simulink model "Controller"  (R2015a)
settings: Solver=ode3  SolverMode=SingleTasking  StartTime=0.0  StopTime=100  FixedStep=T_sim  RelTol=1e-3
PreLoadFcn:
  | LoadLibraries
values from neighbouring files (symbols this model uses):
  a = 10.26    [SetupComplete.m]
  A_x = 0.015    [SetupComplete.m]
  A_y = A_x    (= 0.015)    [SetupComplete.m]
  A_z = 0.16    [SetupComplete.m]
  C_d0 = 0.001193    [SetupComplete.m]
  C_x = 1.2    [SetupComplete.m]
  C_y = C_x    (= 1.2)    [SetupComplete.m]
  C_z = 2.2    [SetupComplete.m]
  CG_0 = [0,0,0.02]'    [SetupComplete.m]
  eta_23 = deg2rad(-1.42)    [Run3Copter.m]
  g = 9.81    [SetupComplete.m]
  h = 0.08    [SetupComplete.m]
  h_M = 0.064    [SetupComplete.m]
  I_BAC_0 = [ Ix,0,Ixz;0,Iy,0;Ixz,0,Iz]    [SetupComplete.m]
  Initial_Omegas = [1;1;1]*Omega_hover    [Run3Copter.m]
  l = 0.3450    (= 0.345)    [NDI_components.m]    (also in SetupComplete.m; robust_controller.m)
  l_arm = 0.264    [SetupComplete.m]
  m = 3.51    [SetupComplete.m]
  m_0 = 2.61    [SetupComplete.m]
  m_M = 0.300    (= 0.3)    [SetupComplete.m]
  R = 0.1778    [SetupComplete.m]    (also in robust_controller.m = eye(4))
  rho = 1.15    [SetupComplete.m]
  sigma = b*c/(pi*R)    (= 0.107416159567)    [SetupComplete.m]
  theta_0 = 0.38397    [SetupComplete.m]
  theta_1 = -0.2967    [SetupComplete.m]
  v_i0 = sqrt( 1/3*m*g/(2*rho*pi*R^2)  )    [SetupComplete.m]
undefined symbols (not defined in the file or in its folder): DOWN_0, EAST_0, Motor, NORTH_0, P_0, Prop, Q_0, R_0, Throttle_Hover, U_0, V_0, v_i_adim, Vx_adim, Vz_adim, W_0
undefined symbols (not defined in the file): Initial_Torques, J_FA, J_T, Rotation_sign, Tau_motors
libraries: XXCopter x39, simulink x35, vrlib x15, simulink_extras x7, aerolib6dofsys x2, qcatlib x2, dspinverses x2
(part 4 of 10)

== system Controller/P Controller/NDI+CA Controller/ 9DOF NDI+CA Controller - No massic update/1st order reference model ==
  y_ref : Inport
  y_meas : Inport  Port=2
  Bandwidth gain : Gain  Gain=Kb
  Bandwidth gain 1 : Gain  Gain=Kb
  Command FF gain : Gain  Gain=fc
  Command_dot FF gain : Gain  Gain=Kf
  Integral gain : Gain  Gain=fi
  Integrator : Integrator
  Integrator1 : Integrator
  Kref gain : Gain  Gain=Kref
  Sum15 : Sum  Inputs=|+-
  Sum16 : Sum  Inputs=++-
  Sum17 : Sum  Inputs=++|
  Sum5 : Sum  Inputs=|+-
  y_des_dot : Outport
  wires:
  Integral gain/1 -> Integrator1/1
  Bandwidth gain 1/1 -> Integral gain/1
  y_ref/1 -> Sum5/1
  Command_dot FF gain/1 -> Sum17/1
  Command FF gain/1 -> Sum16/1
  Integrator/1 -> Command FF gain/1, Sum15/1, Sum5/2  "y_c"
  y_meas/1 -> Sum16/3, Sum15/2
  Sum16/1 -> Bandwidth gain/1
  Kref gain/1 -> Integrator/1, Command_dot FF gain/1  "y_dot_c"
  Integrator1/1 -> Sum16/2
  Sum17/1 -> y_des_dot/1
  Bandwidth gain/1 -> Sum17/2
  Sum15/1 -> Bandwidth gain 1/1
  Sum5/1 -> Kref gain/1

== system Controller/P Controller/NDI+CA Controller/ 9DOF NDI+CA Controller - No massic update/Control Allocation 9DOF ==
  Pseudocontrol input : Inport
  Effectiveness control matrix : Inport  Port=2
  Control Allocation 9DOF : Subsystem  VariantControl=(default)
  Pseudoinverse 9DOF : Subsystem  VariantControl=Variant1
  Control output : Outport

== system Controller/P Controller/NDI+CA Controller/4DOF NDI+CA Controller - No massic update/1st order reference model ==
  y_ref : Inport
  y_meas : Inport  Port=2
  Bandwidth gain : Gain  Gain=Kb
  Bandwidth gain 1 : Gain  Gain=Kb
  Command FF gain : Gain  Gain=fc
  Command_dot FF gain : Gain  Gain=Kf
  Integral gain : Gain  Gain=fi
  Integrator : Integrator
  Integrator1 : Integrator
  Kref gain : Gain  Gain=Kref
  Sum15 : Sum  Inputs=|+-
  Sum16 : Sum  Inputs=++-
  Sum17 : Sum  Inputs=++|
  Sum5 : Sum  Inputs=|+-
  y_des_dot : Outport
  wires:
  Sum5/1 -> Kref gain/1
  Sum15/1 -> Bandwidth gain 1/1
  Bandwidth gain/1 -> Sum17/2
  Sum17/1 -> y_des_dot/1
  Integrator1/1 -> Sum16/2
  Kref gain/1 -> Command_dot FF gain/1, Integrator/1  "y_dot_c"
  Sum16/1 -> Bandwidth gain/1
  y_meas/1 -> Sum15/2, Sum16/3
  Integrator/1 -> Sum5/2, Sum15/1, Command FF gain/1  "y_c"
  Command FF gain/1 -> Sum16/1
  Command_dot FF gain/1 -> Sum17/1
  y_ref/1 -> Sum5/1
  Bandwidth gain 1/1 -> Integral gain/1
  Integral gain/1 -> Integrator1/1

== system Controller/P Controller/NDI+CA Controller/4DOF NDI+CA Controller - No massic update/1st order reference model1 ==
  y_ref : Inport
  y_meas : Inport  Port=2
  Bandwidth gain : Gain  Gain=Kb
  Bandwidth gain 1 : Gain  Gain=Kb
  Command FF gain : Gain  Gain=fc
  Command_dot FF gain : Gain  Gain=Kf
  Integral gain : Gain  Gain=fi
  Integrator : Integrator
  Integrator1 : Integrator
  Kref gain : Gain  Gain=Kref
  Sum15 : Sum  Inputs=|+-
  Sum16 : Sum  Inputs=++-
  Sum17 : Sum  Inputs=++|
  Sum5 : Sum  Inputs=|+-
  y_des_dot : Outport
  wires:
  Sum5/1 -> Kref gain/1
  Sum15/1 -> Bandwidth gain 1/1
  Bandwidth gain/1 -> Sum17/2
  Sum17/1 -> y_des_dot/1
  Integrator1/1 -> Sum16/2
  Kref gain/1 -> Command_dot FF gain/1, Integrator/1  "y_dot_c"
  Sum16/1 -> Bandwidth gain/1
  y_meas/1 -> Sum15/2, Sum16/3
  Integrator/1 -> Sum5/2, Sum15/1, Command FF gain/1  "y_c"
  Command FF gain/1 -> Sum16/1
  Command_dot FF gain/1 -> Sum17/1
  y_ref/1 -> Sum5/1
  Bandwidth gain 1/1 -> Integral gain/1
  Integral gain/1 -> Integrator1/1

== system Controller/P Controller/NDI+CA Controller/4DOF NDI+CA Controller - No massic update/1st order reference model2 ==
  y_ref : Inport
  y_meas : Inport  Port=2
  Bandwidth gain : Gain  Gain=Kb
  Bandwidth gain 1 : Gain  Gain=Kb
  Command FF gain : Gain  Gain=fc
  Command_dot FF gain : Gain  Gain=Kf
  Integral gain : Gain  Gain=fi
  Integrator : Integrator
  Integrator1 : Integrator
  Kref gain : Gain  Gain=Kref
  Sum15 : Sum  Inputs=|+-
  Sum16 : Sum  Inputs=++-
  Sum17 : Sum  Inputs=++|
  Sum5 : Sum  Inputs=|+-
  y_des_dot : Outport
  wires:
  Sum5/1 -> Kref gain/1
  Sum15/1 -> Bandwidth gain 1/1
  Bandwidth gain/1 -> Sum17/2
  Sum17/1 -> y_des_dot/1
  Integrator1/1 -> Sum16/2
  Kref gain/1 -> Command_dot FF gain/1, Integrator/1  "y_dot_c"
  Sum16/1 -> Bandwidth gain/1
  y_meas/1 -> Sum15/2, Sum16/3
  Integrator/1 -> Sum5/2, Sum15/1, Command FF gain/1  "y_c"
  Command FF gain/1 -> Sum16/1
  Command_dot FF gain/1 -> Sum17/1
  y_ref/1 -> Sum5/1
  Bandwidth gain 1/1 -> Integral gain/1
  Integral gain/1 -> Integrator1/1

== system Controller/P Controller/NDI+CA Controller/4DOF NDI+CA Controller - No massic update/1st order reference model3 ==
  y_ref : Inport
  y_meas : Inport  Port=2
  Bandwidth gain : Gain  Gain=Kb
  Bandwidth gain 1 : Gain  Gain=Kb
  Command FF gain : Gain  Gain=fc
  Command_dot FF gain : Gain  Gain=Kf
  Integral gain : Gain  Gain=fi
  Integrator : Integrator
  Integrator1 : Integrator
  Kref gain : Gain  Gain=Kref
  Sum15 : Sum  Inputs=|+-
  Sum16 : Sum  Inputs=++-
  Sum17 : Sum  Inputs=++|
  Sum5 : Sum  Inputs=|+-
  y_des_dot : Outport
  wires:
  Integral gain/1 -> Integrator1/1
  Bandwidth gain 1/1 -> Integral gain/1
  y_ref/1 -> Sum5/1
  Command_dot FF gain/1 -> Sum17/1
  Command FF gain/1 -> Sum16/1
  Integrator/1 -> Command FF gain/1, Sum15/1, Sum5/2  "y_c"
  y_meas/1 -> Sum16/3, Sum15/2
  Sum16/1 -> Bandwidth gain/1
  Kref gain/1 -> Integrator/1, Command_dot FF gain/1  "y_dot_c"
  Integrator1/1 -> Sum16/2
  Sum17/1 -> y_des_dot/1
  Bandwidth gain/1 -> Sum17/2
  Sum15/1 -> Bandwidth gain 1/1
  Sum5/1 -> Kref gain/1

== system Controller/P Controller/NDI+CA Controller/4DOF NDI+CA Controller - No massic update/Control Allocation 4DOF ==
  Pseudocontrol input : Inport
  Effectiveness control matrix : Inport  Port=2
  Control Allocation 4DOF : Subsystem  VariantControl=(default)
  Pseudoinverse : Subsystem  VariantControl=Variant1
  Control output : Outport

== system Controller/P Controller/NDI+CA Controller/9DOF NDI+CA Controller/Mass Properties ==
  Arms DCMs : Inport
  CG_0 : Inport  Port=2
  m_0 : Inport  Port=3
  m : Inport  Port=4
  m_M : Inport  Port=5
  I_BAC_0 : Inport  Port=6
  Arm Inertia : MATLAB Function  TreatAsAtomicUnit=on
  Bus Selector : BusSelector  OutputSignals=T_FaFb1,T_FaFb2,T_FaFb3
  CG position : Sum
  Divide : Product  Inputs=*/
  Divide1 : Product  Inputs=**
  Divide2 : Product  Inputs=/*
  Divide3 : Product  Inputs=**
  Motors Pos sum : Sum  Inputs=+++
  Total I_BAC : Sum
  I_BAC : Outport
  CG : Outport  Port=2
  wires:
  Arms DCMs/1 -> Bus Selector/1
  Bus Selector/3 -> Arm Inertia/3(T3_FAFb)  "<T_FaFb3>"
  Bus Selector/2 -> Arm Inertia/2(T2_FAFb)  "<T_FaFb2>"
  Bus Selector/1 -> Arm Inertia/1(T1_FAFb)  "<T_FaFb1>"
  Total I_BAC/1 -> I_BAC/1
  m_0/1 -> Divide/1
  m/1 -> Divide/2, Divide2/1
  CG_0/1 -> Divide1/1
  Divide/1 -> Divide1/2
  m_M/1 -> Divide2/2
  CG position/1 -> CG/1
  Divide1/1 -> CG position/1
  Motors Pos sum/1 -> Divide3/1
  Divide2/1 -> Divide3/2
  Divide3/1 -> CG position/2
  Arm Inertia/3(r2_M) -> Motors Pos sum/2
  Arm Inertia/4(r3_M) -> Motors Pos sum/1
  Arm Inertia/1(I_M) -> Total I_BAC/2
  I_BAC_0/1 -> Total I_BAC/1
  Arm Inertia/2(r1_M) -> Motors Pos sum/3

== system Controller/3 Copter Complete/Arms Dynamics: Forces and Moments/4 DOF Arms Dynamics: Forces and Moments1/4 DOF Arms Dynamics: Forces and Moments1/Arm Dynamics ==
  note: Motor-Propeller Coupling: Propeller Torque
  Throttle [0-1] : Inport
  Comm Angles (rad) : Inport  Port=2
  Omega_Initial : Inport  Port=3
  h_ground : Inport  Port=4
  omega_b : Inport  Port=5
  V_b : Inport  Port=6
  Aerodynamics Propeller : Subsystem  TreatAsAtomicUnit=on  mask{Rot_sign=Rot_sign}
      mask prompts: Rot_sign "Rotation Sign"
      settings: MinAlgLoopOccurrences=on
      mask TypeOptions Rot_sign: Rotation_sign/Value
  Arms Kinematics : Subsystem  AncestorBlock=XXCopter/Arms Kinematics  TreatAsAtomicUnit=on  mask{Arm_number=arm_num, Arm_hub_position=arm_hub_pos, eta_dir=eta_dir, gamma_dir=gamma_dir, h_prop=h}
      mask prompts: Arm_number "Arm number (1,2 or 3)"; Arm_hub_position "Arm Hub position"; eta_dir "eta direcction"; gamma_dir "gamma diretion"; h_prop "h of propeller hub"
      mask help:
      | If Arm number 1 (Forward one)
      | eta_dir=[1,0,0]
      | gamma_dir=[0,1,0]
      |
      | If Arm number 2 or 3 (rear ones)
      | eta_dir=[0,1,0]
      | gamma_dir=[1,0,0]
      mask TypeOptions Arm_number: Arm_no/Value
      mask TypeOptions Arm_hub_position: Hub_position/Value
      mask TypeOptions eta_dir: eta_dir/Gain
      mask TypeOptions gamma_dir: gamma_dir/Gain
      mask TypeOptions h_prop: h arm/Value
  Cross Product : vrlib/Utilities/Cross Product
  ESC+Motor Dynamcis : XXCopter/ESC+Motor Dynamcis  Inertia_swithc_var=Motor+Prop  J_T=J_T  tau=tau
  Ground : Ground
  Gyroscopic Moments : XXCopter/Gyroscopic Moments  Arm_axis=[l_arm;0;0]  Rot_sign=Rot_sign  eta_dir=eta_dir  gamma_dir=gamma_dir  J_T=J_T  J_FA=J_FA
  Initial_torque : Memory  X0=Torq_ini
  Scope : Scope
      settings: YMin=-25  SaveName=ScopeData10
  Servos Dynamics : Subsystem  AncestorBlock=XXCopter/Servos Dynamics  TreatAsAtomicUnit=on  mask{omega_n=omega_n, xi=xi, derv_param=c, init_eta=init_eta, init_gamma=0}
      mask prompts: omega_n "Servo natural freq (rad/s) omega_n"; xi "Servo damping xi"; derv_param "Derivative parameter"; init_eta "Initial eta (rad)"; init_gamma "Initial gamma (rad)"
      mask TypeOptions init_eta: init_eta/Value | init_eta1/Value
      mask TypeOptions init_gamma: init_gamma/Value | init_gamma1/Value
  Total moments : Sum
  V^A (m/s) : Sum  Inputs=+++
  initial_omega : Memory  X0=Omega_ini
  initial_omega1 : Memory  X0=Omega_ini
  omega_A : Sum
  omega_b1 : InportShadow  Port=5
  Forces : Outport
  Moments : Outport  Port=2
  Omega_out : Outport  Port=3
  Omega_dot_out : Outport  Port=4
  T_FaFb : Outport  Port=5
  Angles (rad) : Outport  Port=6
  r_p : Outport  Port=7
  wires:
  initial_omega/1 -> ESC+Motor Dynamcis/2
  Initial_torque/1 -> ESC+Motor Dynamcis/4
  Aerodynamics Propeller/1(Prop_Torque_out) -> Initial_torque/1
  Total moments/1 -> Moments/1
  Gyroscopic Moments/1 -> Total moments/2
  Aerodynamics Propeller/3(Moments_prop @Fb) -> Total moments/1
  Ground/1 -> Servos Dynamics/2(Torques?)
  Servos Dynamics/3(Angles_dot_dot (rad/s^2)) -> Gyroscopic Moments/5
  omega_A/1 -> Gyroscopic Moments/2
  omega_b1/1 -> omega_A/2, Gyroscopic Moments/3
  Arms Kinematics/4(omega_Ab (rad/s)) -> omega_A/1
  Servos Dynamics/2(Angles_dot (rad/s)) -> Arms Kinematics/2(Angles_dot (rad/s)), Gyroscopic Moments/4
  Aerodynamics Propeller/2(Forces_prop @Fb) -> Scope/1, Forces/1
  Arms Kinematics/1(r_p (m)) -> r_p/1, Cross Product/2, Aerodynamics Propeller/3(r_p)
  Arms Kinematics/3(T_F_a,Fb) -> T_FaFb/1, Aerodynamics Propeller/5(T_FaFb), Gyroscopic Moments/1
  V^A (m/s)/1 -> Aerodynamics Propeller/4(V^A)
  Arms Kinematics/2(r_p_dot (m/s)) -> V^A (m/s)/3
  V_b/1 -> V^A (m/s)/1
  Cross Product/1 -> V^A (m/s)/2
  omega_b/1 -> Cross Product/1
  Servos Dynamics/1(Angles Arms (rad)) -> Angles (rad)/1, Arms Kinematics/1(Angles (rad))
  Comm Angles (rad)/1 -> Servos Dynamics/1(Com Angles (rad))
  h_ground/1 -> Aerodynamics Propeller/2(h_ground)
  ESC+Motor Dynamcis/1 -> Aerodynamics Propeller/1(Omega), Omega_out/1, Gyroscopic Moments/6, initial_omega/1  "Omega"
  ESC+Motor Dynamcis/2 -> Omega_dot_out/1, Gyroscopic Moments/7  "Omega_dot"
  Omega_Initial/1 -> ESC+Motor Dynamcis/3
  Throttle [0-1]/1 -> ESC+Motor Dynamcis/1

== system Controller/3 Copter Complete/Arms Dynamics: Forces and Moments/4 DOF Arms Dynamics: Forces and Moments1/4 DOF Arms Dynamics: Forces and Moments1/Arm Dynamics1 ==
  note: Motor-Propeller Coupling: Propeller Torque
  Throttle [0-1] : Inport
  Comm Angles (rad) : Inport  Port=2
  Omega_Initial : Inport  Port=3
  h_ground : Inport  Port=4
  omega_b : Inport  Port=5
  V_b : Inport  Port=6
  Aerodynamics Propeller : Subsystem  TreatAsAtomicUnit=on  mask{Rot_sign=Rot_sign}
      mask prompts: Rot_sign "Rotation Sign"
      settings: MinAlgLoopOccurrences=on
      mask TypeOptions Rot_sign: Rotation_sign/Value
  Arms Kinematics : Subsystem  AncestorBlock=XXCopter/Arms Kinematics  TreatAsAtomicUnit=on  mask{Arm_number=arm_num, Arm_hub_position=arm_hub_pos, eta_dir=eta_dir, gamma_dir=gamma_dir, h_prop=h}
      mask prompts: Arm_number "Arm number (1,2 or 3)"; Arm_hub_position "Arm Hub position"; eta_dir "eta direcction"; gamma_dir "gamma diretion"; h_prop "h of propeller hub"
      mask help:
      | If Arm number 1 (Forward one)
      | eta_dir=[1,0,0]
      | gamma_dir=[0,1,0]
      |
      | If Arm number 2 or 3 (rear ones)
      | eta_dir=[0,1,0]
      | gamma_dir=[1,0,0]
      mask TypeOptions Arm_number: Arm_no/Value
      mask TypeOptions Arm_hub_position: Hub_position/Value
      mask TypeOptions eta_dir: eta_dir/Gain
      mask TypeOptions gamma_dir: gamma_dir/Gain
      mask TypeOptions h_prop: h arm/Value
  Cross Product : vrlib/Utilities/Cross Product
  Display : Display
  ESC+Motor Dynamcis : XXCopter/ESC+Motor Dynamcis  Inertia_swithc_var=Motor+Prop  J_T=J_T  tau=tau
  Ground : Ground
  Gyroscopic Moments : XXCopter/Gyroscopic Moments  Arm_axis=[0;l_arm;0]  Rot_sign=Rot_sign  eta_dir=eta_dir  gamma_dir=gamma_dir  J_T=J_T  J_FA=J_FA
  Initial_torque : Memory  X0=Torq_ini
  Scope : Scope
      settings: YMin=-30  YMax=10  SaveName=ScopeData11
  Scope1 : Scope
      settings: YMin=-1.5  YMax=1  SaveName=ScopeData12
  Servos Dynamics : XXCopter/Servos Dynamics  omega_n=omega_n  xi=xi  derv_param=c  init_eta=init_eta  init_gamma=0
      link override eta_1: Numerator=0  Denominator=1
      link override eta_2: Numerator=0  Denominator=1
  Total moments : Sum
  V^A (m/s) : Sum  Inputs=+++
  initial_omega : Memory  X0=Omega_ini
  omega_A : Sum
  omega_b1 : InportShadow  Port=5
  Forces : Outport
  Moments : Outport  Port=2
  Omega_out : Outport  Port=3
  Omega_dot_out : Outport  Port=4
  T_FaFb : Outport  Port=5
  Angles (rad) : Outport  Port=6
  r_p : Outport  Port=7
  wires:
  initial_omega/1 -> ESC+Motor Dynamcis/2
  Initial_torque/1 -> ESC+Motor Dynamcis/4
  Aerodynamics Propeller/1(Prop_Torque_out) -> Initial_torque/1
  Total moments/1 -> Moments/1
  Gyroscopic Moments/1 -> Total moments/2
  Aerodynamics Propeller/3(Moments_prop @Fb) -> Total moments/1
  Ground/1 -> Servos Dynamics/2
  Servos Dynamics/3 -> Gyroscopic Moments/5
  omega_A/1 -> Gyroscopic Moments/2
  omega_b1/1 -> omega_A/2, Gyroscopic Moments/3
  Arms Kinematics/4(omega_Ab (rad/s)) -> omega_A/1
  Servos Dynamics/2 -> Arms Kinematics/2(Angles_dot (rad/s)), Gyroscopic Moments/4
  Aerodynamics Propeller/2(Forces_prop @Fb) -> Scope/1, Forces/1
  Arms Kinematics/1(r_p (m)) -> r_p/1, Cross Product/2, Aerodynamics Propeller/3(r_p)
  Arms Kinematics/3(T_F_a,Fb) -> T_FaFb/1, Aerodynamics Propeller/5(T_FaFb), Display/1, Gyroscopic Moments/1
  V^A (m/s)/1 -> Scope1/1, Aerodynamics Propeller/4(V^A)
  Arms Kinematics/2(r_p_dot (m/s)) -> V^A (m/s)/3
  V_b/1 -> V^A (m/s)/1
  Cross Product/1 -> V^A (m/s)/2
  omega_b/1 -> Cross Product/1
  Servos Dynamics/1 -> Angles (rad)/1, Arms Kinematics/1(Angles (rad))
  Comm Angles (rad)/1 -> Servos Dynamics/1
  h_ground/1 -> Aerodynamics Propeller/2(h_ground)
  ESC+Motor Dynamcis/1 -> Aerodynamics Propeller/1(Omega), Omega_out/1, Gyroscopic Moments/6, initial_omega/1  "Omega"
  ESC+Motor Dynamcis/2 -> Omega_dot_out/1, Gyroscopic Moments/7  "Omega_dot"
  Omega_Initial/1 -> ESC+Motor Dynamcis/3
  Throttle [0-1]/1 -> ESC+Motor Dynamcis/1

== system Controller/3 Copter Complete/Arms Dynamics: Forces and Moments/4 DOF Arms Dynamics: Forces and Moments1/4 DOF Arms Dynamics: Forces and Moments1/Arm Dynamics2 ==
  note: Motor-Propeller Coupling: Propeller Torque
  Throttle [0-1] : Inport
  Comm Angles (rad) : Inport  Port=2
  Omega_Initial : Inport  Port=3
  h_ground : Inport  Port=4
  omega_b : Inport  Port=5
  V_b : Inport  Port=6
  Aerodynamics Propeller : Subsystem  TreatAsAtomicUnit=on  mask{Rot_sign=Rot_sign}
      mask prompts: Rot_sign "Rotation Sign"
      settings: MinAlgLoopOccurrences=on
      mask TypeOptions Rot_sign: Rotation_sign/Value
  Arms Kinematics : Subsystem  AncestorBlock=XXCopter/Arms Kinematics  TreatAsAtomicUnit=on  mask{Arm_number=arm_num, Arm_hub_position=arm_hub_pos, eta_dir=eta_dir, gamma_dir=gamma_dir, h_prop=h}
      mask prompts: Arm_number "Arm number (1,2 or 3)"; Arm_hub_position "Arm Hub position"; eta_dir "eta direcction"; gamma_dir "gamma diretion"; h_prop "h of propeller hub"
      mask help:
      | If Arm number 1 (Forward one)
      | eta_dir=[1,0,0]
      | gamma_dir=[0,1,0]
      |
      | If Arm number 2 or 3 (rear ones)
      | eta_dir=[0,1,0]
      | gamma_dir=[1,0,0]
      mask TypeOptions Arm_number: Arm_no/Value
      mask TypeOptions Arm_hub_position: Hub_position/Value
      mask TypeOptions eta_dir: eta_dir/Gain
      mask TypeOptions gamma_dir: gamma_dir/Gain
      mask TypeOptions h_prop: h arm/Value
  Cross Product : vrlib/Utilities/Cross Product
  ESC+Motor Dynamcis : XXCopter/ESC+Motor Dynamcis  Inertia_swithc_var=Motor+Prop  J_T=J_T  tau=tau
  Ground : Ground
  Gyroscopic Moments : XXCopter/Gyroscopic Moments  Arm_axis=[0;-l_arm;0]  Rot_sign=Rot_sign  eta_dir=eta_dir  gamma_dir=gamma_dir  J_T=J_T  J_FA=J_FA
  Initial_torque : Memory  X0=Torq_ini
  Servos Dynamics : Subsystem  AncestorBlock=XXCopter/Servos Dynamics  TreatAsAtomicUnit=on  mask{omega_n=omega_n, xi=xi, derv_param=c, init_eta=init_eta, init_gamma=0}
      mask prompts: omega_n "Servo natural freq (rad/s) omega_n"; xi "Servo damping xi"; derv_param "Derivative parameter"; init_eta "Initial eta (rad)"; init_gamma "Initial gamma (rad)"
      mask TypeOptions init_eta: init_eta/Value | init_eta1/Value
      mask TypeOptions init_gamma: init_gamma/Value | init_gamma1/Value
  Total moments : Sum
  V^A (m/s) : Sum  Inputs=+++
  initial_omega : Memory  X0=Omega_ini
  omega_A : Sum
  omega_b1 : InportShadow  Port=5
  Forces : Outport
  Moments : Outport  Port=2
  Omega_out : Outport  Port=3
  Omega_dot_out : Outport  Port=4
  T_FaFb : Outport  Port=5
  Angles (rad) : Outport  Port=6
  r_p : Outport  Port=7
  wires:
  initial_omega/1 -> ESC+Motor Dynamcis/2
  Initial_torque/1 -> ESC+Motor Dynamcis/4
  Aerodynamics Propeller/1(Prop_Torque_out) -> Initial_torque/1
  Total moments/1 -> Moments/1
  Gyroscopic Moments/1 -> Total moments/2
  Aerodynamics Propeller/3(Moments_prop @Fb) -> Total moments/1
  Ground/1 -> Servos Dynamics/2(Torques?)
  Servos Dynamics/3(Angles_dot_dot (rad/s^2)) -> Gyroscopic Moments/5
  omega_A/1 -> Gyroscopic Moments/2
  omega_b1/1 -> omega_A/2, Gyroscopic Moments/3
  Arms Kinematics/4(omega_Ab (rad/s)) -> omega_A/1
  Servos Dynamics/2(Angles_dot (rad/s)) -> Arms Kinematics/2(Angles_dot (rad/s)), Gyroscopic Moments/4
  Aerodynamics Propeller/2(Forces_prop @Fb) -> Forces/1
  Arms Kinematics/1(r_p (m)) -> r_p/1, Cross Product/2, Aerodynamics Propeller/3(r_p)
  Arms Kinematics/3(T_F_a,Fb) -> T_FaFb/1, Aerodynamics Propeller/5(T_FaFb), Gyroscopic Moments/1
  V^A (m/s)/1 -> Aerodynamics Propeller/4(V^A)
  Arms Kinematics/2(r_p_dot (m/s)) -> V^A (m/s)/3
  V_b/1 -> V^A (m/s)/1
  Cross Product/1 -> V^A (m/s)/2
  omega_b/1 -> Cross Product/1
  Servos Dynamics/1(Angles Arms (rad)) -> Angles (rad)/1, Arms Kinematics/1(Angles (rad))
  Comm Angles (rad)/1 -> Servos Dynamics/1(Com Angles (rad))
  h_ground/1 -> Aerodynamics Propeller/2(h_ground)
  ESC+Motor Dynamcis/1 -> Aerodynamics Propeller/1(Omega), Omega_out/1, Gyroscopic Moments/6, initial_omega/1  "Omega"
  ESC+Motor Dynamcis/2 -> Omega_dot_out/1, Gyroscopic Moments/7  "Omega_dot"
  Omega_Initial/1 -> ESC+Motor Dynamcis/3
  Throttle [0-1]/1 -> ESC+Motor Dynamcis/1

== system Controller/3 Copter Complete/Arms Dynamics: Forces and Moments/9 DOF Arms Dynamics: Forces and Moments/9 DOF Arms Dynamics: Forces and Moments/Arm Dynamics ==
  note: Motor-Propeller Coupling: Propeller Torque
  Throttle [0-1] : Inport
  Comm Angles (rad) : Inport  Port=2
  Omega_Initial : Inport  Port=3
  h_ground : Inport  Port=4
  omega_b : Inport  Port=5
  V_b : Inport  Port=6
  Aerodynamics Propeller : Subsystem  TreatAsAtomicUnit=on  mask{Rot_sign=Rot_sign}
      mask prompts: Rot_sign "Rotation Sign"
      settings: MinAlgLoopOccurrences=on
      mask TypeOptions Rot_sign: Rotation_sign/Value
  Arms Kinematics : XXCopter/Arms Kinematics  Arm_number=arm_num  Arm_hub_position=arm_hub_pos  eta_dir=eta_dir  gamma_dir=gamma_dir  h_prop=h
  Cross Product : vrlib/Utilities/Cross Product
  ESC+Motor Dynamcis : XXCopter/ESC+Motor Dynamcis  Inertia_swithc_var=Motor+Prop  J_T=J_T  tau=tau
  Ground : Ground
  Gyroscopic Moments : XXCopter/Gyroscopic Moments  Arm_axis=[l_arm;0;0]  Rot_sign=Rot_sign  eta_dir=eta_dir  gamma_dir=gamma_dir  J_T=J_T  J_FA=J_FA
  Initial_torque : Memory  X0=Torq_ini
  Servos Dynamics : XXCopter/Servos Dynamics  omega_n=omega_n  xi=xi  derv_param=c  init_eta=init_eta  init_gamma=0
  Total moments : Sum
  V^A (m/s) : Sum  Inputs=+++
  initial_omega : Memory  X0=Omega_ini
  omega_A : Sum
  omega_b1 : InportShadow  Port=5
  Forces : Outport
  Moments : Outport  Port=2
  Omega_out : Outport  Port=3
  Omega_dot_out : Outport  Port=4
  T_FaFb : Outport  Port=5
  Angles (rad) : Outport  Port=6
  r_p : Outport  Port=7
  wires:
  initial_omega/1 -> ESC+Motor Dynamcis/2
  Initial_torque/1 -> ESC+Motor Dynamcis/4
  Aerodynamics Propeller/1(Prop_Torque_out) -> Initial_torque/1
  Total moments/1 -> Moments/1
  Gyroscopic Moments/1 -> Total moments/2
  Aerodynamics Propeller/3(Moments_prop @Fb) -> Total moments/1
  Ground/1 -> Servos Dynamics/2
  Servos Dynamics/3 -> Gyroscopic Moments/5
  omega_A/1 -> Gyroscopic Moments/2
  omega_b1/1 -> omega_A/2, Gyroscopic Moments/3
  Arms Kinematics/4 -> omega_A/1
  Servos Dynamics/2 -> Arms Kinematics/2, Gyroscopic Moments/4
  Aerodynamics Propeller/2(Forces_prop @Fb) -> Forces/1
  Arms Kinematics/1 -> r_p/1, Cross Product/2, Aerodynamics Propeller/3(r_p)
  Arms Kinematics/3 -> T_FaFb/1, Aerodynamics Propeller/5(T_FaFb), Gyroscopic Moments/1
  V^A (m/s)/1 -> Aerodynamics Propeller/4(V^A)
  Arms Kinematics/2 -> V^A (m/s)/3
  V_b/1 -> V^A (m/s)/1
  Cross Product/1 -> V^A (m/s)/2
  omega_b/1 -> Cross Product/1
  Servos Dynamics/1 -> Angles (rad)/1, Arms Kinematics/1
  Comm Angles (rad)/1 -> Servos Dynamics/1
  h_ground/1 -> Aerodynamics Propeller/2(h_ground)
  ESC+Motor Dynamcis/1 -> Aerodynamics Propeller/1(Omega), Omega_out/1, Gyroscopic Moments/6, initial_omega/1  "Omega"
  ESC+Motor Dynamcis/2 -> Omega_dot_out/1, Gyroscopic Moments/7  "Omega_dot"
  Omega_Initial/1 -> ESC+Motor Dynamcis/3
  Throttle [0-1]/1 -> ESC+Motor Dynamcis/1

== system Controller/3 Copter Complete/Arms Dynamics: Forces and Moments/9 DOF Arms Dynamics: Forces and Moments/9 DOF Arms Dynamics: Forces and Moments/Arm Dynamics1 ==
  note: Motor-Propeller Coupling: Propeller Torque
  Throttle [0-1] : Inport
  Comm Angles (rad) : Inport  Port=2
  Omega_Initial : Inport  Port=3
  h_ground : Inport  Port=4
  omega_b : Inport  Port=5
  V_b : Inport  Port=6
  Aerodynamics Propeller : Subsystem  TreatAsAtomicUnit=on  mask{Rot_sign=Rot_sign}
      mask prompts: Rot_sign "Rotation Sign"
      settings: MinAlgLoopOccurrences=on
      mask TypeOptions Rot_sign: Rotation_sign/Value
  Arms Kinematics : XXCopter/Arms Kinematics  Arm_number=arm_num  Arm_hub_position=arm_hub_pos  eta_dir=eta_dir  gamma_dir=gamma_dir  h_prop=h
  Cross Product : vrlib/Utilities/Cross Product
  ESC+Motor Dynamcis : XXCopter/ESC+Motor Dynamcis  Inertia_swithc_var=Motor+Prop  J_T=J_T  tau=tau
  Ground : Ground
  Gyroscopic Moments : XXCopter/Gyroscopic Moments  Arm_axis=[0;l_arm;0]  Rot_sign=Rot_sign  eta_dir=eta_dir  gamma_dir=gamma_dir  J_T=J_T  J_FA=J_FA
  Initial_torque : Memory  X0=Torq_ini
  Servos Dynamics : XXCopter/Servos Dynamics  omega_n=omega_n  xi=xi  derv_param=c  init_eta=init_eta  init_gamma=0
  Total moments : Sum
  V^A (m/s) : Sum  Inputs=+++
  initial_omega : Memory  X0=Omega_ini
  omega_A : Sum
  omega_b1 : InportShadow  Port=5
  Forces : Outport
  Moments : Outport  Port=2
  Omega_out : Outport  Port=3
  Omega_dot_out : Outport  Port=4
  T_FaFb : Outport  Port=5
  Angles (rad) : Outport  Port=6
  r_p : Outport  Port=7
  wires:
  initial_omega/1 -> ESC+Motor Dynamcis/2
  Initial_torque/1 -> ESC+Motor Dynamcis/4
  Aerodynamics Propeller/1(Prop_Torque_out) -> Initial_torque/1
  Total moments/1 -> Moments/1
  Gyroscopic Moments/1 -> Total moments/2
  Aerodynamics Propeller/3(Moments_prop @Fb) -> Total moments/1
  Ground/1 -> Servos Dynamics/2
  Servos Dynamics/3 -> Gyroscopic Moments/5
  omega_A/1 -> Gyroscopic Moments/2
  omega_b1/1 -> omega_A/2, Gyroscopic Moments/3
  Arms Kinematics/4 -> omega_A/1
  Servos Dynamics/2 -> Arms Kinematics/2, Gyroscopic Moments/4
  Aerodynamics Propeller/2(Forces_prop @Fb) -> Forces/1
  Arms Kinematics/1 -> r_p/1, Cross Product/2, Aerodynamics Propeller/3(r_p)
  Arms Kinematics/3 -> T_FaFb/1, Aerodynamics Propeller/5(T_FaFb), Gyroscopic Moments/1
  V^A (m/s)/1 -> Aerodynamics Propeller/4(V^A)
  Arms Kinematics/2 -> V^A (m/s)/3
  V_b/1 -> V^A (m/s)/1
  Cross Product/1 -> V^A (m/s)/2
  omega_b/1 -> Cross Product/1
  Servos Dynamics/1 -> Angles (rad)/1, Arms Kinematics/1
  Comm Angles (rad)/1 -> Servos Dynamics/1
  h_ground/1 -> Aerodynamics Propeller/2(h_ground)
  ESC+Motor Dynamcis/1 -> Aerodynamics Propeller/1(Omega), Omega_out/1, Gyroscopic Moments/6, initial_omega/1  "Omega"
  ESC+Motor Dynamcis/2 -> Omega_dot_out/1, Gyroscopic Moments/7  "Omega_dot"
  Omega_Initial/1 -> ESC+Motor Dynamcis/3
  Throttle [0-1]/1 -> ESC+Motor Dynamcis/1

== system Controller/3 Copter Complete/Arms Dynamics: Forces and Moments/9 DOF Arms Dynamics: Forces and Moments/9 DOF Arms Dynamics: Forces and Moments/Arm Dynamics2 ==
  note: Motor-Propeller Coupling: Propeller Torque
  Throttle [0-1] : Inport
  Comm Angles (rad) : Inport  Port=2
  Omega_Initial : Inport  Port=3
  h_ground : Inport  Port=4
  omega_b : Inport  Port=5
  V_b : Inport  Port=6
  Aerodynamics Propeller : Subsystem  TreatAsAtomicUnit=on  mask{Rot_sign=Rot_sign}
      mask prompts: Rot_sign "Rotation Sign"
      settings: MinAlgLoopOccurrences=on
      mask TypeOptions Rot_sign: Rotation_sign/Value
  Arms Kinematics : XXCopter/Arms Kinematics  Arm_number=arm_num  Arm_hub_position=arm_hub_pos  eta_dir=eta_dir  gamma_dir=gamma_dir  h_prop=h
  Cross Product : vrlib/Utilities/Cross Product
  ESC+Motor Dynamcis : XXCopter/ESC+Motor Dynamcis  Inertia_swithc_var=Motor+Prop  J_T=J_T  tau=tau
  Ground : Ground
  Gyroscopic Moments : XXCopter/Gyroscopic Moments  Arm_axis=[0;-l_arm;0]  Rot_sign=Rot_sign  eta_dir=eta_dir  gamma_dir=gamma_dir  J_T=J_T  J_FA=J_FA
  Initial_torque : Memory  X0=Torq_ini
  Servos Dynamics : XXCopter/Servos Dynamics  omega_n=omega_n  xi=xi  derv_param=c  init_eta=init_eta  init_gamma=0
  Total moments : Sum
  V^A (m/s) : Sum  Inputs=+++
  initial_omega : Memory  X0=Omega_ini
  omega_A : Sum
  omega_b1 : InportShadow  Port=5
  Forces : Outport
  Moments : Outport  Port=2
  Omega_out : Outport  Port=3
  Omega_dot_out : Outport  Port=4
  T_FaFb : Outport  Port=5
  Angles (rad) : Outport  Port=6
  r_p : Outport  Port=7
  wires:
  initial_omega/1 -> ESC+Motor Dynamcis/2
  Initial_torque/1 -> ESC+Motor Dynamcis/4
  Aerodynamics Propeller/1(Prop_Torque_out) -> Initial_torque/1
  Total moments/1 -> Moments/1
  Gyroscopic Moments/1 -> Total moments/2
  Aerodynamics Propeller/3(Moments_prop @Fb) -> Total moments/1
  Ground/1 -> Servos Dynamics/2
  Servos Dynamics/3 -> Gyroscopic Moments/5
  omega_A/1 -> Gyroscopic Moments/2
  omega_b1/1 -> omega_A/2, Gyroscopic Moments/3
  Arms Kinematics/4 -> omega_A/1
  Servos Dynamics/2 -> Arms Kinematics/2, Gyroscopic Moments/4
  Aerodynamics Propeller/2(Forces_prop @Fb) -> Forces/1
  Arms Kinematics/1 -> r_p/1, Cross Product/2, Aerodynamics Propeller/3(r_p)
  Arms Kinematics/3 -> T_FaFb/1, Aerodynamics Propeller/5(T_FaFb), Gyroscopic Moments/1
  V^A (m/s)/1 -> Aerodynamics Propeller/4(V^A)
  Arms Kinematics/2 -> V^A (m/s)/3
  V_b/1 -> V^A (m/s)/1
  Cross Product/1 -> V^A (m/s)/2
  omega_b/1 -> Cross Product/1
  Servos Dynamics/1 -> Angles (rad)/1, Arms Kinematics/1
  Comm Angles (rad)/1 -> Servos Dynamics/1
  h_ground/1 -> Aerodynamics Propeller/2(h_ground)
  ESC+Motor Dynamcis/1 -> Aerodynamics Propeller/1(Omega), Omega_out/1, Gyroscopic Moments/6, initial_omega/1  "Omega"
  ESC+Motor Dynamcis/2 -> Omega_dot_out/1, Gyroscopic Moments/7  "Omega_dot"
  Omega_Initial/1 -> ESC+Motor Dynamcis/3
  Throttle [0-1]/1 -> ESC+Motor Dynamcis/1

== system Controller/P Controller/NDI+CA Controller/ 9DOF NDI+CA Controller - No massic update/Control Allocation 9DOF/Control Allocation 9DOF ==
  note: Enabler override saturations and override
      | them with zero to avoid actuators being
      | locked by control allocation algorithm
  note: Weights used to normalize different
      | inputs between controllers.
      | Throttle - 0 to 1
      | Servo - 0 to 2*pi
  note: Position and rate limits for
      | tricopter actuators
  Pseudocontrol input : Inport
  Effectiveness control matrix : Inport  Port=2
  "Control allocator Completed " : qcatlib/Control allocator Completed   alg=WLS  CA_type=QP  iter_max=100  gamma=1e6  k_B=6  m_B=9  T=0.01  tol=0
  Control desired (0 to minimize control effort) : Constant  Value=zeros(1,9)
  Control positions deviation Weight W1 : Constant  Value=diag(1./[1,2*pi,2*pi,1,2*pi,2*pi,1,2*pi,2*pi] )
  Control rate deviation Weight W2 : Constant  Value=diag(1./[1,2*pi,2*pi,1,2*pi,2*pi,1,2*pi,2*pi] )
  Enalbe/Disable : Constant
  Error Weight Wv2 : Constant  Value=blkdiag(1,1,1, 1/(2*pi), 1/(2*pi), 1/(2*pi))
  Position limits 9DOF : Constant  Value=[ [0,-deg2rad(165),-deg2rad(90),0,-deg2rad(165),-deg2rad(15),0,-deg2rad(165),-deg2rad(90)]', [1,deg2rad(165),deg2rad(15),1,deg2rad(165),deg2rad(90),1,deg2rad(165),deg2rad(15)]']
  Rates limits 9DOF : Constant  Value=[ [-17,-1,-1,-17,-1,-1,-17,-1,-1]', [17,1,1,17,1,1,17,1,1]']*1
  Reshape1 : Reshape  OutputDimensionality=Customize  OutputDimensions=[6,9]
  Reshape2 : Reshape  OutputDimensions=[6,1]
  Terminator : Terminator
  Terminator1 : Terminator
  Unit Delay : UnitDelay  SampleTime=-1
  manual Initial saturations : Constant  Value=zeros(9,1)
  Control output : Outport  PortDimensions=9
  wires:
  "Control allocator Completed "/2 -> Terminator/1
  "Control allocator Completed "/3 -> Terminator1/1
  Effectiveness control matrix/1 -> Reshape1/1
  Reshape1/1 -> "Control allocator Completed "/4
  Control desired (0 to minimize control effort)/1 -> "Control allocator Completed "/3
  Position limits 9DOF/1 -> "Control allocator Completed "/5
  Rates limits 9DOF/1 -> "Control allocator Completed "/6
  Error Weight Wv2/1 -> "Control allocator Completed "/7
  Control positions deviation Weight W1/1 -> "Control allocator Completed "/8
  Control rate deviation Weight W2/1 -> "Control allocator Completed "/9
  manual Initial saturations/1 -> "Control allocator Completed "/10
  Enalbe/Disable/1 -> "Control allocator Completed "/11
  Reshape2/1 -> Control output/1
  "Control allocator Completed "/1 -> Reshape2/1, Unit Delay/1
  Unit Delay/1 -> "Control allocator Completed "/2
  Pseudocontrol input/1 -> "Control allocator Completed "/1

== system Controller/P Controller/NDI+CA Controller/ 9DOF NDI+CA Controller - No massic update/Control Allocation 9DOF/Pseudoinverse 9DOF ==
  Pseudocontrol input : Inport
  Effectiveness control matrix : Inport  Port=2
  Product1 : Product  Multiplication=Matrix(*)
  Pseudoinverse : dspinverses/Pseudoinverse  wanterr=off
  Reshape1 : Reshape  OutputDimensions=[6,1]
  Control output : Outport  PortDimensions=9
  wires:
  Product1/1 -> Reshape1/1
  Pseudoinverse/1 -> Product1/1
  Effectiveness control matrix/1 -> Pseudoinverse/1
  Pseudocontrol input/1 -> Product1/2
  Reshape1/1 -> Control output/1

== system Controller/P Controller/NDI+CA Controller/4DOF NDI+CA Controller - No massic update/Control Allocation 4DOF/Control Allocation 4DOF ==
  note: Position and rate limits for
      | tricopter actuators
  note: Weights used to normalize different
      | inputs between controllers.
      | Throttle - 0 to 1
      | Servo - 0 to 2*pi
  note: Enabler override saturations and override
      | them with zero to avoid actuators being
      | locked by control allocation algorithm
  Pseudocontrol input : Inport
  Effectiveness control matrix : Inport  Port=2
  "Control allocator Completed " : qcatlib/Control allocator Completed   alg=WLS  CA_type=QP  iter_max=100  gamma=1e6  k_B=4  m_B=4  T=0.01  tol=0
  Control desired (0 to minimize control effort) : Constant  Value=zeros(1,4)
  Control positions deviation Weight W1 : Constant  Value=diag(1./[1,2*pi,1,1] )
  Control rate deviation Weight W2 : Constant  Value=diag(1./[1,2*pi,1,1] )
  Demux : Demux
  Enalbe/Disable : Constant
  Error Weight Wv2 : Constant  Value=blkdiag(1, 1/(2*pi), 1/(2*pi), 1/(2*pi))
  Ground{,1..4} (5 alike) : Ground
  Mux10 : Mux  Inputs=9
  Position limits 4 DOF : Constant  Value=[ [0,-deg2rad(165),0,0]', [1,deg2rad(160),1,1]']
  Rates limits 4DOF : Constant  Value=[ [-17,-1,-17,-17]', [17,1,17,17]']*1
  Reshape1 : Reshape  OutputDimensionality=Customize  OutputDimensions=[4,4]
  Reshape2 : Reshape  OutputDimensions=[6,1]
  Terminator : Terminator
  Terminator1 : Terminator
  Unit Delay : UnitDelay  SampleTime=-1
  manual Initial saturations : Constant  Value=zeros(4,1)
  Control output : Outport  PortDimensions=9
  wires:
  Pseudocontrol input/1 -> "Control allocator Completed "/1
  Unit Delay/1 -> "Control allocator Completed "/2
  "Control allocator Completed "/1 -> Unit Delay/1, Demux/1
  Ground4/1 -> Mux10/9
  Ground3/1 -> Mux10/8
  Ground2/1 -> Mux10/6
  Ground1/1 -> Mux10/5
  Ground/1 -> Mux10/3
  Demux/4 -> Mux10/7
  Demux/3 -> Mux10/4
  Demux/2 -> Mux10/2
  Demux/1 -> Mux10/1
  Mux10/1 -> Reshape2/1
  Reshape2/1 -> Control output/1
  Enalbe/Disable/1 -> "Control allocator Completed "/11
  manual Initial saturations/1 -> "Control allocator Completed "/10
  Control rate deviation Weight W2/1 -> "Control allocator Completed "/9
  Control positions deviation Weight W1/1 -> "Control allocator Completed "/8
  Error Weight Wv2/1 -> "Control allocator Completed "/7
  Rates limits 4DOF/1 -> "Control allocator Completed "/6
  Position limits 4 DOF/1 -> "Control allocator Completed "/5
  Control desired (0 to minimize control effort)/1 -> "Control allocator Completed "/3
  Reshape1/1 -> "Control allocator Completed "/4
  Effectiveness control matrix/1 -> Reshape1/1
  "Control allocator Completed "/3 -> Terminator1/1
  "Control allocator Completed "/2 -> Terminator/1

== system Controller/P Controller/NDI+CA Controller/4DOF NDI+CA Controller - No massic update/Control Allocation 4DOF/Pseudoinverse ==
  Pseudocontrol input : Inport
  Effectiveness control matrix : Inport  Port=2
  Demux : Demux
  Ground{,1..4} (5 alike) : Ground
  Mux10 : Mux  Inputs=9
  Product1 : Product  Multiplication=Matrix(*)
  Pseudoinverse : dspinverses/Pseudoinverse  wanterr=off
  Reshape1 : Reshape  OutputDimensions=[6,1]
  Control output : Outport  PortDimensions=9
  wires:
  Reshape1/1 -> Control output/1
  Pseudocontrol input/1 -> Product1/2
  Effectiveness control matrix/1 -> Pseudoinverse/1
  Pseudoinverse/1 -> Product1/1
  Mux10/1 -> Reshape1/1
  Demux/1 -> Mux10/1
  Demux/2 -> Mux10/2
  Demux/3 -> Mux10/4
  Demux/4 -> Mux10/7
  Ground/1 -> Mux10/3
  Ground1/1 -> Mux10/5
  Ground2/1 -> Mux10/6
  Ground3/1 -> Mux10/8
  Ground4/1 -> Mux10/9
  Product1/1 -> Demux/1

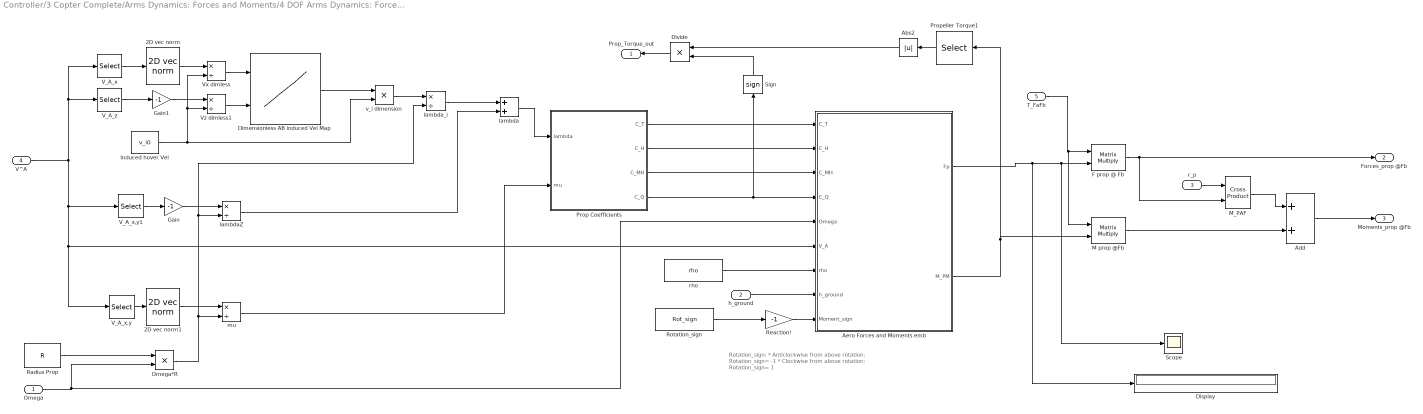
== system Controller/3 Copter Complete/Arms Dynamics: Forces and Moments/4 DOF Arms Dynamics: Forces and Moments1/4 DOF Arms Dynamics: Forces and Moments1/Arm Dynamics/Aerodynamics Propeller ==
  note: Rotation_sign:
      |
      | * Anticlockwise from above rotation: Rotation_sign= -1
      | * Clockwise from above rotation: Rotation_sign= 1
  Omega : Inport
  h_ground : Inport  Port=2
  r_p : Inport  Port=3
  V^A : Inport  Port=4
  T_FaFb : Inport  Port=5
  2D vec norm : XXCopter/2D vec norm
  2D vec norm1 : XXCopter/2D vec norm
  Abs2 : Abs
  Add : Sum
  Aero Forces and Moments emb : Subsystem  AncestorBlock=XXCopter/Aero Forces and Moments emb  TreatAsAtomicUnit=on
  Dimensionless AB induced Vel Map : Lookup_n-D  BreakpointsForDimension1=Vx_adim  BreakpointsForDimension2=Vz_adim  BreakpointsForDimension3=[5, 7]  Table=v_i_adim  RndMeth=Simplest  InputSameDT=on
  Display : Display
  Divide : Product  Inputs=**
  F prop @ Fb : Product  Multiplication=Matrix(*)
  Gain : Gain  Gain=-1
  Gain1 : Gain  Gain=-1
  Induced hover Vel : Constant  Value=v_i0
  M prop @Fb : Product  Multiplication=Matrix(*)
  M_PAF : vrlib/Utilities/Cross Product
  Omega*R : Product  Inputs=**
  Prop Coefficients : MATLAB Function  TreatAsAtomicUnit=on
  Propeller Torque1 : Selector  IndexMode=Zero-based  InputPortWidth=3  Indices=2
  Radius Prop : Constant  Value=R
  Reaction! : Gain  Gain=-1
  Rotation_sign : Constant  Value=Rot_sign
  Scope : Scope
      settings: YMin=-20  YMax=2.5  SaveName=ScopeData9
  Sign : Signum
  V_A_x : Selector  InputPortWidth=3  Indices=[1 2]
  V_A_x,y : Selector  InputPortWidth=3  Indices=[1 2]
  V_A_x,y1 : Selector  InputPortWidth=3  Indices=[3]
  V_A_z : Selector  InputPortWidth=3  Indices=3
  Vx dimless : Product  Inputs=*/
  Vz dimless1 : Product  Inputs=*/
  lambda : Sum
  lambdaZ : Product  Inputs=*/
  lambda_i : Product  Inputs=*/
  mu : Product  Inputs=*/
  rho : Constant  Value=rho
  v_i dimension : Product  Inputs=**
  Prop_Torque_out : Outport
  Forces_prop @Fb : Outport  Port=2
  Moments_prop @Fb : Outport  Port=3
  wires:
  Abs2/1 -> Divide/1
  Sign/1 -> Divide/2
  Propeller Torque1/1 -> Abs2/1
  Divide/1 -> Prop_Torque_out/1
  rho/1 -> Aero Forces and Moments emb/7(rho)
  Reaction!/1 -> Aero Forces and Moments emb/9(Moment_sign)
  Prop Coefficients/4(C_Q) -> Aero Forces and Moments emb/4(C_Q), Sign/1
  mu/1 -> Prop Coefficients/2(mu)
  2D vec norm/1 -> Vx dimless/1
  M prop @Fb/1 -> Add/2
  M_PAF/1 -> Add/1
  r_p/1 -> M_PAF/1
  F prop @ Fb/1 -> Forces_prop @Fb/1, M_PAF/2
  Aero Forces and Moments emb/1(Fp) -> Display/1, Scope/1, F prop @ Fb/2
  T_FaFb/1 -> F prop @ Fb/1, M prop @Fb/1
  Rotation_sign/1 -> Reaction!/1
  h_ground/1 -> Aero Forces and Moments emb/8(h_ground)
  Add/1 -> Moments_prop @Fb/1
  Aero Forces and Moments emb/2("M_PM ") -> Propeller Torque1/1, M prop @Fb/2
  Omega/1 -> Omega*R/2, Aero Forces and Moments emb/5(Omega)
  V^A/1 -> V_A_z/1, V_A_x/1, V_A_x,y1/1, Aero Forces and Moments emb/6(V_A), V_A_x,y/1
  Prop Coefficients/3(C_MH) -> Aero Forces and Moments emb/3(C_MH)
  Prop Coefficients/2(C_H) -> Aero Forces and Moments emb/2(C_H)
  Prop Coefficients/1(C_T) -> Aero Forces and Moments emb/1(C_T)
  lambda/1 -> Prop Coefficients/1(lambda)
  Gain1/1 -> Vz dimless1/1
  lambdaZ/1 -> lambda/2
  lambda_i/1 -> lambda/1
  Gain/1 -> lambdaZ/1
  V_A_x,y1/1 -> Gain/1
  v_i dimension/1 -> lambda_i/1
  Dimensionless AB induced Vel Map/1 -> v_i dimension/1
  Induced hover Vel/1 -> Vx dimless/2, Vz dimless1/2, v_i dimension/2
  V_A_z/1 -> Gain1/1
  Vz dimless1/1 -> Dimensionless AB induced Vel Map/2
  V_A_x/1 -> 2D vec norm/1
  Vx dimless/1 -> Dimensionless AB induced Vel Map/1
  Omega*R/1 -> lambda_i/2, lambdaZ/2, mu/2
  2D vec norm1/1 -> mu/1
  V_A_x,y/1 -> 2D vec norm1/1
  Radius Prop/1 -> Omega*R/1

== system Controller/3 Copter Complete/Arms Dynamics: Forces and Moments/4 DOF Arms Dynamics: Forces and Moments1/4 DOF Arms Dynamics: Forces and Moments1/Arm Dynamics/Arms Kinematics ==
  Angles (rad) : Inport
  Angles_dot (rad/s) : Inport  Port=2
  Add : Sum
  Add3 : Sum
  Arm_no : Constant  Value=Arm_number
  Cross Product : vrlib/Utilities/Cross Product
  DCM Arm : MATLAB Function  TreatAsAtomicUnit=on
  Demux : Demux  Outputs=2
  Demux3 : Demux  Outputs=2
  Fa->Fb : Product  Multiplication=Matrix(*)
  Gain7 : Gain  Gain=[0;0;-1]
  Hub_position : Constant  Value=Arm_hub_position
  Matrix Multiply : Product  Multiplication=Matrix(*)
  Permute Dimensions : PermuteDimensions
  eta_dir : Gain  Gain=eta_dir
  gamma_dir : Gain  Gain=gamma_dir
  h arm : Constant  Value=h_prop
  r_p (m) : Outport
  r_p_dot (m/s) : Outport  Port=2
  T_F_a,Fb : Outport  Port=3
  omega_Ab (rad/s) : Outport  Port=4
  wires:
  Arm_no/1 -> DCM Arm/1(arm_no)
  Cross Product/1 -> r_p_dot (m/s)/1
  Fa->Fb/1 -> Add3/2, Cross Product/2
  Hub_position/1 -> Add3/1
  Gain7/1 -> Fa->Fb/2
  h arm/1 -> Gain7/1
  Add3/1 -> r_p (m)/1  "r_p (m)"
  Add/1 -> omega_Ab (rad/s)/1, Cross Product/1  "omega_Ab"
  eta_dir/1 -> Add/1
  Matrix Multiply/1 -> Add/2
  gamma_dir/1 -> Matrix Multiply/2
  Demux3/1 -> eta_dir/1  "eta_dot"
  Demux3/2 -> gamma_dir/1  "gamma_dot"
  Angles_dot (rad/s)/1 -> Demux3/1
  Demux/2 -> DCM Arm/3(gamma)
  Demux/1 -> DCM Arm/2(eta)
  Angles (rad)/1 -> Demux/1
  Permute Dimensions/1 -> Fa->Fb/1, Matrix Multiply/1, T_F_a,Fb/1  "T_F_a,Fb"
  DCM Arm/1(T_Fb_FA) -> Permute Dimensions/1

== system Controller/3 Copter Complete/Arms Dynamics: Forces and Moments/4 DOF Arms Dynamics: Forces and Moments1/4 DOF Arms Dynamics: Forces and Moments1/Arm Dynamics/Servos Dynamics ==
  Com Angles (rad) : Inport
  Torques? : Inport  Port=2
  Add : Sum  Inputs=+-
  Add1 : Sum
  Demux : Demux  Outputs=2
  Derivative{,1..3} (4 alike) : Derivative  CoefficientInTFapproximation=derv_param
  Mux{,1..4} (5 alike) : Mux  Inputs=2
  Terminator : Terminator
  eta_1 : TransferFcn  Numerator=omega_n^2  Denominator=[1 xi*omega_n omega_n^2]
  gamma_1 : TransferFcn  Numerator=0  Denominator=1
  init_eta : Constant  Value=init_eta
  init_eta1 : Constant  Value=init_eta
  init_gamma : Constant  Value=init_gamma
  init_gamma1 : Constant  Value=init_gamma
  Angles Arms (rad) : Outport
  Angles_dot (rad/s) : Outport  Port=2
  Angles_dot_dot (rad/s^2) : Outport  Port=3
  wires:
  Add1/1 -> Angles Arms (rad)/1
  Mux4/1 -> Add1/1
  Mux/1 -> Add1/2
  init_gamma1/1 -> Mux4/2
  init_eta1/1 -> Mux4/1
  init_gamma/1 -> Mux3/2
  Mux3/1 -> Add/2
  init_eta/1 -> Mux3/1
  Add/1 -> Demux/1
  Torques?/1 -> Terminator/1
  Derivative/1 -> Derivative2/1, Mux1/1
  Derivative3/1 -> Mux2/2
  Derivative2/1 -> Mux2/1
  Derivative1/1 -> Mux1/2, Derivative3/1
  Mux2/1 -> Angles_dot_dot (rad/s^2)/1
  Mux1/1 -> Angles_dot (rad/s)/1
  gamma_1/1 -> Derivative1/1, Mux/2
  eta_1/1 -> Mux/1, Derivative/1
  Demux/2 -> gamma_1/1
  Demux/1 -> eta_1/1
  Com Angles (rad)/1 -> Add/1

== system Controller/3 Copter Complete/Arms Dynamics: Forces and Moments/4 DOF Arms Dynamics: Forces and Moments1/4 DOF Arms Dynamics: Forces and Moments1/Arm Dynamics1/Aerodynamics Propeller ==
  note: Rotation_sign:
      |
      | * Anticlockwise from above rotation: Rotation_sign= -1
      | * Clockwise from above rotation: Rotation_sign= 1
  Omega : Inport
  h_ground : Inport  Port=2
  r_p : Inport  Port=3
  V^A : Inport  Port=4
  T_FaFb : Inport  Port=5
  2D vec norm : XXCopter/2D vec norm
  2D vec norm1 : XXCopter/2D vec norm
  Abs2 : Abs
  Add : Sum
  Aero Forces and Moments emb : Subsystem  AncestorBlock=XXCopter/Aero Forces and Moments emb  TreatAsAtomicUnit=on
  Dimensionless AB induced Vel Map : Lookup_n-D  BreakpointsForDimension1=Vx_adim  BreakpointsForDimension2=Vz_adim  BreakpointsForDimension3=[5, 7]  Table=v_i_adim  RndMeth=Simplest  InputSameDT=on
  Divide : Product  Inputs=**
  F prop @ Fb : Product  Multiplication=Matrix(*)
  Gain : Gain  Gain=-1
  Gain1 : Gain  Gain=-1
  Induced hover Vel : Constant  Value=v_i0
  M prop @Fb : Product  Multiplication=Matrix(*)
  M_PAF : vrlib/Utilities/Cross Product
  Omega*R : Product  Inputs=**
  Prop Coefficients : MATLAB Function  TreatAsAtomicUnit=on
  Propeller Torque1 : Selector  IndexMode=Zero-based  InputPortWidth=3  Indices=2
  Radius Prop : Constant  Value=R
  Reaction! : Gain  Gain=-1
  Rotation_sign : Constant  Value=Rot_sign
  Sign : Signum
  V_A_x : Selector  InputPortWidth=3  Indices=[1 2]
  V_A_x,y : Selector  InputPortWidth=3  Indices=[1 2]
  V_A_x,y1 : Selector  InputPortWidth=3  Indices=[3]
  V_A_z : Selector  InputPortWidth=3  Indices=3
  Vx dimless : Product  Inputs=*/
  Vz dimless1 : Product  Inputs=*/
  lambda : Sum
  lambdaZ : Product  Inputs=*/
  lambda_i : Product  Inputs=*/
  mu : Product  Inputs=*/
  rho : Constant  Value=rho
  v_i dimension : Product  Inputs=**
  Prop_Torque_out : Outport
  Forces_prop @Fb : Outport  Port=2
  Moments_prop @Fb : Outport  Port=3
  wires:
  Abs2/1 -> Divide/1
  Sign/1 -> Divide/2
  Propeller Torque1/1 -> Abs2/1
  Divide/1 -> Prop_Torque_out/1
  rho/1 -> Aero Forces and Moments emb/7(rho)
  Reaction!/1 -> Aero Forces and Moments emb/9(Moment_sign)
  Prop Coefficients/4(C_Q) -> Aero Forces and Moments emb/4(C_Q), Sign/1
  mu/1 -> Prop Coefficients/2(mu)
  2D vec norm/1 -> Vx dimless/1
  M prop @Fb/1 -> Add/2
  M_PAF/1 -> Add/1
  r_p/1 -> M_PAF/1
  F prop @ Fb/1 -> Forces_prop @Fb/1, M_PAF/2
  Aero Forces and Moments emb/1(Fp) -> F prop @ Fb/2
  T_FaFb/1 -> F prop @ Fb/1, M prop @Fb/1
  Rotation_sign/1 -> Reaction!/1
  h_ground/1 -> Aero Forces and Moments emb/8(h_ground)
  Add/1 -> Moments_prop @Fb/1
  Aero Forces and Moments emb/2("M_PM ") -> Propeller Torque1/1, M prop @Fb/2
  Omega/1 -> Omega*R/2, Aero Forces and Moments emb/5(Omega)
  V^A/1 -> V_A_z/1, V_A_x/1, V_A_x,y1/1, Aero Forces and Moments emb/6(V_A), V_A_x,y/1
  Prop Coefficients/3(C_MH) -> Aero Forces and Moments emb/3(C_MH)
  Prop Coefficients/2(C_H) -> Aero Forces and Moments emb/2(C_H)
  Prop Coefficients/1(C_T) -> Aero Forces and Moments emb/1(C_T)
  lambda/1 -> Prop Coefficients/1(lambda)
  Gain1/1 -> Vz dimless1/1
  lambdaZ/1 -> lambda/2
  lambda_i/1 -> lambda/1
  Gain/1 -> lambdaZ/1
  V_A_x,y1/1 -> Gain/1
  v_i dimension/1 -> lambda_i/1
  Dimensionless AB induced Vel Map/1 -> v_i dimension/1
  Induced hover Vel/1 -> Vx dimless/2, Vz dimless1/2, v_i dimension/2
  V_A_z/1 -> Gain1/1
  Vz dimless1/1 -> Dimensionless AB induced Vel Map/2
  V_A_x/1 -> 2D vec norm/1
  Vx dimless/1 -> Dimensionless AB induced Vel Map/1
  Omega*R/1 -> lambda_i/2, lambdaZ/2, mu/2
  2D vec norm1/1 -> mu/1
  V_A_x,y/1 -> 2D vec norm1/1
  Radius Prop/1 -> Omega*R/1

== system Controller/3 Copter Complete/Arms Dynamics: Forces and Moments/4 DOF Arms Dynamics: Forces and Moments1/4 DOF Arms Dynamics: Forces and Moments1/Arm Dynamics1/Arms Kinematics ==
  Angles (rad) : Inport
  Angles_dot (rad/s) : Inport  Port=2
  Add : Sum
  Add3 : Sum
  Arm_no : Constant  Value=Arm_number
  Cross Product : vrlib/Utilities/Cross Product
  DCM Arm : MATLAB Function  TreatAsAtomicUnit=on
  Demux : Demux  Outputs=2
  Demux3 : Demux  Outputs=2
  Fa->Fb : Product  Multiplication=Matrix(*)
  Gain7 : Gain  Gain=[0;0;-1]
  Hub_position : Constant  Value=Arm_hub_position
  Matrix Multiply : Product  Multiplication=Matrix(*)
  Permute Dimensions : PermuteDimensions
  eta_dir : Gain  Gain=eta_dir
  gamma_dir : Gain  Gain=gamma_dir
  h arm : Constant  Value=h_prop
  r_p (m) : Outport
  r_p_dot (m/s) : Outport  Port=2
  T_F_a,Fb : Outport  Port=3
  omega_Ab (rad/s) : Outport  Port=4
  wires:
  Arm_no/1 -> DCM Arm/1(arm_no)
  Cross Product/1 -> r_p_dot (m/s)/1
  Fa->Fb/1 -> Add3/2, Cross Product/2
  Hub_position/1 -> Add3/1
  Gain7/1 -> Fa->Fb/2
  h arm/1 -> Gain7/1
  Add3/1 -> r_p (m)/1  "r_p (m)"
  Add/1 -> omega_Ab (rad/s)/1, Cross Product/1  "omega_Ab"
  eta_dir/1 -> Add/1
  Matrix Multiply/1 -> Add/2
  gamma_dir/1 -> Matrix Multiply/2
  Demux3/1 -> eta_dir/1  "eta_dot"
  Demux3/2 -> gamma_dir/1  "gamma_dot"
  Angles_dot (rad/s)/1 -> Demux3/1
  Demux/2 -> DCM Arm/3(gamma)
  Demux/1 -> DCM Arm/2(eta)
  Angles (rad)/1 -> Demux/1
  Permute Dimensions/1 -> Fa->Fb/1, Matrix Multiply/1, T_F_a,Fb/1  "T_F_a,Fb"
  DCM Arm/1(T_Fb_FA) -> Permute Dimensions/1
